simulink model "Mooventure2016_Rev5"  (Simulink 7.7)
settings: Solver=FixedStepDiscrete  StartTime=0.0  StopTime=10  RelTol=1e-3
PreLoadFcn:
  | try, eval([bdroot '_setup']); catch, eval('model_setup', ''); end
InitFcn:
  | try, eval([bdroot '_setup']); catch, eval('model_setup', ''); end
undefined symbols (not defined in the file): ECM, H1, motohawk_build_version, motohawk_trunc_name, motohawk_vardec_config_group, motohawk_vardec_path, xD
libraries: MotoHawk_lib x976, motohawk_control_primitives_lib x41, simulink x27, motohawk_annotations_lib x3
(part 13 of 16)

== system Mooventure2016_Rev5/Foreground/Control/Faults/Accesories/HV-Heater System ==
  In1 : Inport
  Abs : Abs
  Add : Sum
  Add1 : Sum  Inputs=+-
  Bus Selector : BusSelector  OutputSignals=Analog_Inputs.Coolant.temp_reading
  Bus Selector1 : BusSelector  OutputSignals=Analog_Inputs.Coolant.temp_reading
  Bus Selector2 : BusSelector  OutputSignals=Analog_Inputs.Coolant.Heater_Temp_Raw
  Bus Selector3 : BusSelector  OutputSignals=Analog_Inputs.Coolant.Heater_Temp_Raw
  Bus Selector4 : BusSelector  OutputSignals=Analog_Inputs.Coolant.Heater_Temp_Raw
  Logical Operator : Logic  Operator=OR  Inputs=4  AllPortsSameDT=off  OutDataTypeStr=boolean
  Logical Operator1 : Logic  Operator=NOT  AllPortsSameDT=off  OutDataTypeStr=boolean
  Logical Operator2 : Logic  AllPortsSameDT=off  OutDataTypeStr=boolean
  Relational Operator : RelationalOperator  OutDataTypeStr=boolean
  Relational Operator1 : RelationalOperator  Operator=>  OutDataTypeStr=boolean
  Relational Operator2 : RelationalOperator  OutDataTypeStr=boolean
  Relational Operator3 : RelationalOperator  Operator=<  OutDataTypeStr=boolean
  Relational Operator4 : RelationalOperator  Operator=>  OutDataTypeStr=boolean
  Triggered Subsystem : Subsystem  TreatAsAtomicUnit=on
  Unit Delay : UnitDelay  SampleTime=-1
  motohawk_calibration : MotoHawk_lib/Calibration & Probing Blocks/motohawk_calibration  nam='Temp_Fault_Hyst'  val=4  storage=Calibration  show_more=off  name_source=Use Parameter  data_type=Inherit from 'Default Value'  read_level=1  write_level=1  ovr_cals=on  view_as=Number  enum_struct={'Disabled', 'Enabled'}  vector_style=Wide Row  use_help_units=off  help=''  units=''  use_header_enum=off  row_header_enum={}  col_header_enum={}  use_min_max=off  min_val=-inf  max_val=inf  use_precision=off  precision=''  gain=1  offset=0  exp=1  use_mototune_group=off  mototune_group=motohawk_vardec_path(gcb)
  motohawk_calibration1 : MotoHawk_lib/Calibration & Probing Blocks/motohawk_calibration  nam='HV_Heater_Over_Temperature_Fault'  val=93  storage=Calibration  show_more=off  name_source=Use Parameter  data_type=Inherit from 'Default Value'  read_level=1  write_level=1  ovr_cals=on  view_as=Number  enum_struct={'Disabled', 'Enabled'}  vector_style=Wide Row  use_help_units=off  help=''  units=''  use_header_enum=off  row_header_enum={}  col_header_enum={}  use_min_max=off  min_val=-inf  max_val=inf  use_precision=off  precision=''  gain=1  offset=0  exp=1  use_mototune_group=off  mototune_group=motohawk_vardec_path(gcb)
  motohawk_calibration2 : MotoHawk_lib/Calibration & Probing Blocks/motohawk_calibration  nam='HV_Heater_Temperature_Sensor_A_Intermittent_Fault'  val=4  storage=Calibration  show_more=off  name_source=Use Parameter  data_type=Inherit from 'Default Value'  read_level=1  write_level=1  ovr_cals=on  view_as=Number  enum_struct={'Disabled', 'Enabled'}  vector_style=Wide Row  use_help_units=off  help=''  units=''  use_header_enum=off  row_header_enum={}  col_header_enum={}  use_min_max=off  min_val=-inf  max_val=inf  use_precision=off  precision=''  gain=1  offset=0  exp=1  use_mototune_group=off  mototune_group=motohawk_vardec_path(gcb)
  motohawk_calibration3 : MotoHawk_lib/Calibration & Probing Blocks/motohawk_calibration  nam='HV_Heater_Temperature_Sensor_A_Low_Voltage_Fault'  val=20  storage=Calibration  show_more=off  name_source=Use Parameter  data_type=Inherit from 'Default Value'  read_level=1  write_level=1  ovr_cals=on  view_as=Number  enum_struct={'Disabled', 'Enabled'}  vector_style=Wide Row  use_help_units=off  help=''  units=''  use_header_enum=off  row_header_enum={}  col_header_enum={}  use_min_max=off  min_val=-inf  max_val=inf  use_precision=off  precision=''  gain=1  offset=0  exp=1  use_mototune_group=off  mototune_group=motohawk_vardec_path(gcb)
  motohawk_calibration4 : MotoHawk_lib/Calibration & Probing Blocks/motohawk_calibration  nam='HV_Heater_Temperature_Sensor_A_High_Voltage_Fault'  val=250  storage=Calibration  show_more=off  name_source=Use Parameter  data_type=Inherit from 'Default Value'  read_level=1  write_level=1  ovr_cals=on  view_as=Number  enum_struct={'Disabled', 'Enabled'}  vector_style=Wide Row  use_help_units=off  help=''  units=''  use_header_enum=off  row_header_enum={}  col_header_enum={}  use_min_max=off  min_val=-inf  max_val=inf  use_precision=off  precision=''  gain=1  offset=0  exp=1  use_mototune_group=off  mototune_group=motohawk_vardec_path(gcb)
  motohawk_data_def : MotoHawk_lib/Data Storage Blocks/motohawk_data_def  nam='TempReading'  container_nam=''  data=23  typ=double  struct_nam='MyStruct'  storage=Volatile  outputRef=off  use_vardec=off  window=Display  read_level=1  write_level=1  ovr_cals=on  view_as=Number  enum_struct={'Disabled', 'Enabled'}  vector_style=Wide Row  use_help_units=off  help=''  units=''  use_header_enum=off  row_header_enum=''  col_header_enum=''  use_min_max=off  min_val=-inf  max_val=inf  use_precision=off  precision=''  gain=1  offset=0  exp=1  use_mototune_group=off  mototune_group=motohawk_vardec_path(gcb)  eval_name=MyData  data_stores=motohawk_sfun_data_def_data_stores  struct_instances=motohawk_sfun_data_def_struct_instances  vardecs=motohawk_sfun_data_def_vardecs
  motohawk_data_read : MotoHawk_lib/Data Storage Blocks/motohawk_data_read  source=Lookup By Name  structure=Scalar  operation=Read scalar from location by index  sz_vec=4  sz_row=2  sz_col=3  typ=double  nam='TempReading'  checkNull=on  struct_inst_name='MyData'  struct_nam='MyStruct'
  motohawk_fault_def1 : MotoHawk_lib/Fault Management Blocks/motohawk_fault_def  nam='HV_Heater_Poor_Performance'  mode=Enabled  id=['B1B30']  x=1500  y=2000  input_suspected=on  indeterminate=off  increment_xy=on  downsample_count=1  ovr_cals=on  ovr_actions=on  show_actions=on  action1_name=''  action1_cond=(None)  action2_name=''  action2_cond=(None)  action3_name=''  action3_cond=(None)  action4_name=''  action4_cond=(None)
  motohawk_fault_def2 : MotoHawk_lib/Fault Management Blocks/motohawk_fault_def  nam='HV_Heater_Over_Temperature'  mode=Enabled  id=['B1B31']  x=9  y=10  input_suspected=on  indeterminate=off  increment_xy=on  downsample_count=1  ovr_cals=on  ovr_actions=on  show_actions=on  action1_name=''  action1_cond=(None)  action2_name=''  action2_cond=(None)  action3_name=''  action3_cond=(None)  action4_name=''  action4_cond=(None)
  motohawk_fault_def3 : MotoHawk_lib/Fault Management Blocks/motohawk_fault_def  nam='HV_Heater_Temperature_Sensor_A_Intermittent'  mode=Enabled  id=['B1B32']  x=9  y=10  input_suspected=on  indeterminate=off  increment_xy=on  downsample_count=1  ovr_cals=on  ovr_actions=on  show_actions=on  action1_name=''  action1_cond=(None)  action2_name=''  action2_cond=(None)  action3_name=''  action3_cond=(None)  action4_name=''  action4_cond=(None)
  motohawk_fault_def4 : MotoHawk_lib/Fault Management Blocks/motohawk_fault_def  nam='HV_Heater_Temperature_Sensor_A_Low_Voltage'  mode=Enabled  id=['B1B33']  x=9  y=10  input_suspected=on  indeterminate=off  increment_xy=on  downsample_count=1  ovr_cals=on  ovr_actions=on  show_actions=on  action1_name=''  action1_cond=(None)  action2_name=''  action2_cond=(None)  action3_name=''  action3_cond=(None)  action4_name=''  action4_cond=(None)
  motohawk_fault_def5 : MotoHawk_lib/Fault Management Blocks/motohawk_fault_def  nam='HV_Heater_Temperature_Sensor_A_High_Voltage'  mode=Enabled  id=['B1B34']  x=9  y=10  input_suspected=on  indeterminate=off  increment_xy=on  downsample_count=1  ovr_cals=on  ovr_actions=on  show_actions=on  action1_name=''  action1_cond=(None)  action2_name=''  action2_cond=(None)  action3_name=''  action3_cond=(None)  action4_name=''  action4_cond=(None)
  wires:
  In1/1 -> Bus Selector/1, Bus Selector1/1, Bus Selector2/1, Bus Selector3/1, Bus Selector4/1
  [Heat1] -> Logical Operator/1
  [Heat2] -> Logical Operator/2
  [Heat3] -> Logical Operator/3
  [Heat4] -> Logical Operator/4
  Bus Selector/1 -> Triggered Subsystem/1(In1), Add/2  "<temp_reading>"
  Logical Operator/1 -> Triggered Subsystem/Trigger, Logical Operator2/2
  motohawk_calibration/1 -> Add/1
  Add/1 -> Relational Operator/1
  motohawk_data_read/1 -> Relational Operator/2
  Relational Operator/1 -> Logical Operator1/1
  Logical Operator1/1 -> Logical Operator2/1
  Logical Operator2/1 -> motohawk_fault_def1/1
  motohawk_calibration1/1 -> Relational Operator1/2
  Relational Operator1/1 -> motohawk_fault_def2/1
  Bus Selector1/1 -> Relational Operator1/1  "<temp_reading>"
  Bus Selector2/1 -> Add1/1, Unit Delay/1  "<Heater_Temp_Raw>"
  Unit Delay/1 -> Add1/2
  Add1/1 -> Abs/1
  Abs/1 -> Relational Operator2/1
  Relational Operator2/1 -> motohawk_fault_def3/1
  motohawk_calibration2/1 -> Relational Operator2/2
  motohawk_calibration3/1 -> Relational Operator3/2
  Relational Operator3/1 -> motohawk_fault_def4/1
  Bus Selector3/1 -> Relational Operator3/1  "<Heater_Temp_Raw>"
  motohawk_calibration4/1 -> Relational Operator4/2
  Relational Operator4/1 -> motohawk_fault_def5/1
  Bus Selector4/1 -> Relational Operator4/1  "<Heater_Temp_Raw>"

== system Mooventure2016_Rev5/Foreground/Control/Faults/Battery/2G BMS & Comms ==
  In1 : Inport
  Add : Sum  Inputs=+-
  Bus Selector1 : BusSelector  OutputSignals=Battery_Inputs.CellBalanceingActive
  Bus Selector2 : BusSelector  OutputSignals=Battery_Inputs.ActiveDTC
  Bus Selector3 : BusSelector  OutputSignals=Battery_Inputs.BatteryCurrent
  Bus Selector4 : BusSelector  OutputSignals=Battery_Inputs.AgeCount
  Bus Selector5 : BusSelector  OutputSignals=Battery_Inputs.MaxCellVoltage,Battery_Inputs.MinCellVoltage
  Bus Selector6 : BusSelector  OutputSignals=Battery_Inputs.StateOfCharge
  Bus Selector7 : BusSelector  OutputSignals=Battery_Inputs.BatteryVoltage
  Logical Operator : Logic  AllPortsSameDT=off  OutDataTypeStr=boolean
  Relational Operator{1..3,6} (4 alike) : RelationalOperator  Operator=>  OutDataTypeStr=boolean
  Relational Operator4 : RelationalOperator  OutDataTypeStr=boolean
  Relational Operator5 : RelationalOperator  Operator===  OutDataTypeStr=boolean
  motohawk_calibration1 : MotoHawk_lib/Calibration & Probing Blocks/motohawk_calibration  nam='HV_Battery_2G_BMS_Fault'  val=0  storage=Calibration  show_more=off  name_source=Use Parameter  data_type=Inherit from 'Default Value'  read_level=1  write_level=1  ovr_cals=on  view_as=Number  enum_struct={'Disabled', 'Enabled'}  vector_style=Wide Row  use_help_units=off  help=''  units=''  use_header_enum=off  row_header_enum={}  col_header_enum={}  use_min_max=off  min_val=-inf  max_val=inf  use_precision=off  precision=''  gain=1  offset=0  exp=1  use_mototune_group=off  mototune_group=motohawk_vardec_path(gcb)
  motohawk_calibration2 : MotoHawk_lib/Calibration & Probing Blocks/motohawk_calibration  nam='HV_Battery_Cell_Balancing_Required_Fault'  val=0.3  storage=Calibration  show_more=off  name_source=Use Parameter  data_type=Inherit from 'Default Value'  read_level=1  write_level=1  ovr_cals=on  view_as=Number  enum_struct={'Disabled', 'Enabled'}  vector_style=Wide Row  use_help_units=off  help=''  units=''  use_header_enum=off  row_header_enum={}  col_header_enum={}  use_min_max=off  min_val=-inf  max_val=inf  use_precision=off  precision=''  gain=1  offset=0  exp=1  use_mototune_group=off  mototune_group=motohawk_vardec_path(gcb)
  motohawk_calibration3 : MotoHawk_lib/Calibration & Probing Blocks/motohawk_calibration  nam='HV_Battery_Try_To_Balance_Under_Load_Fault'  val=1  storage=Calibration  show_more=off  name_source=Use Parameter  data_type=Inherit from 'Default Value'  read_level=1  write_level=1  ovr_cals=on  view_as=Number  enum_struct={'Disabled', 'Enabled'}  vector_style=Wide Row  use_help_units=off  help=''  units=''  use_header_enum=off  row_header_enum={}  col_header_enum={}  use_min_max=off  min_val=-inf  max_val=inf  use_precision=off  precision=''  gain=1  offset=0  exp=1  use_mototune_group=off  mototune_group=motohawk_vardec_path(gcb)
  motohawk_calibration4 : MotoHawk_lib/Calibration & Probing Blocks/motohawk_calibration  nam='HV_Battery_48_Controller_Communication_Fault'  val=1000  storage=Calibration  show_more=off  name_source=Use Parameter  data_type=Inherit from 'Default Value'  read_level=1  write_level=1  ovr_cals=on  view_as=Number  enum_struct={'Disabled', 'Enabled'}  vector_style=Wide Row  use_help_units=off  help=''  units=''  use_header_enum=off  row_header_enum={}  col_header_enum={}  use_min_max=off  min_val=-inf  max_val=inf  use_precision=off  precision=''  gain=1  offset=0  exp=1  use_mototune_group=off  mototune_group=motohawk_vardec_path(gcb)
  motohawk_calibration5 : MotoHawk_lib/Calibration & Probing Blocks/motohawk_calibration  nam='HV_Battery_Too_Low_For_Load_Fault'  val=0  storage=Calibration  show_more=off  name_source=Use Parameter  data_type=Inherit from 'Default Value'  read_level=1  write_level=1  ovr_cals=on  view_as=Number  enum_struct={'Disabled', 'Enabled'}  vector_style=Wide Row  use_help_units=off  help=''  units=''  use_header_enum=off  row_header_enum={}  col_header_enum={}  use_min_max=off  min_val=-inf  max_val=inf  use_precision=off  precision=''  gain=1  offset=0  exp=1  use_mototune_group=off  mototune_group=motohawk_vardec_path(gcb)
  motohawk_calibration6 : MotoHawk_lib/Calibration & Probing Blocks/motohawk_calibration  nam='HV_Battery_Above_Safe_Charge_Point'  val=395  storage=Calibration  show_more=off  name_source=Use Parameter  data_type=Inherit from 'Default Value'  read_level=1  write_level=1  ovr_cals=on  view_as=Number  enum_struct={'Disabled', 'Enabled'}  vector_style=Wide Row  use_help_units=off  help=''  units=''  use_header_enum=off  row_header_enum={}  col_header_enum={}  use_min_max=off  min_val=-inf  max_val=inf  use_precision=off  precision=''  gain=1  offset=0  exp=1  use_mototune_group=off  mototune_group=motohawk_vardec_path(gcb)
  motohawk_fault_def1 : MotoHawk_lib/Fault Management Blocks/motohawk_fault_def  nam='HV_Battery_2G_BMS_Fault'  mode=Enabled  id=['B1C47']  x=9  y=10  input_suspected=on  indeterminate=off  increment_xy=on  downsample_count=1  ovr_cals=on  ovr_actions=on  show_actions=on  action1_name='HV_Light'  action1_cond=Active  action2_name=''  action2_cond=(None)  action3_name=''  action3_cond=(None)  action4_name=''  action4_cond=(None)
  motohawk_fault_def2 : MotoHawk_lib/Fault Management Blocks/motohawk_fault_def  nam='HV_Battery_Too_Low_For_Load'  mode=Enabled  id=['B1C4A']  x=1500  y=2000  input_suspected=on  indeterminate=off  increment_xy=on  downsample_count=1  ovr_cals=on  ovr_actions=on  show_actions=on  action1_name='HV_Light'  action1_cond=Active  action2_name=''  action2_cond=(None)  action3_name=''  action3_cond=(None)  action4_name=''  action4_cond=(None)
  motohawk_fault_def3 : MotoHawk_lib/Fault Management Blocks/motohawk_fault_def  nam='HV_Battery_Try_To_Balance_Under_Load'  mode=Enabled  id=['B1C48']  x=9  y=10  input_suspected=on  indeterminate=off  increment_xy=on  downsample_count=1  ovr_cals=on  ovr_actions=on  show_actions=on  action1_name=''  action1_cond=(None)  action2_name=''  action2_cond=(None)  action3_name=''  action3_cond=(None)  action4_name=''  action4_cond=(None)
  motohawk_fault_def4 : MotoHawk_lib/Fault Management Blocks/motohawk_fault_def  nam='HV_Battery_Cell_Balancing_Required_Fault'  mode=Disabled  id=['B1C49']  x=9  y=10  input_suspected=on  indeterminate=off  increment_xy=on  downsample_count=1  ovr_cals=on  ovr_actions=on  show_actions=on  action1_name='HV_Light'  action1_cond=Active  action2_name=''  action2_cond=(None)  action3_name=''  action3_cond=(None)  action4_name=''  action4_cond=(None)
  motohawk_fault_def5 : MotoHawk_lib/Fault Management Blocks/motohawk_fault_def  nam='HV_Battery_48_Controller_Communication_Fault'  mode=Enabled  id=['B1C50']  x=5  y=10  input_suspected=on  indeterminate=off  increment_xy=on  downsample_count=1  ovr_cals=on  ovr_actions=on  show_actions=on  action1_name='HV_Light'  action1_cond=Active  action2_name='Dyno_Shutdown'  action2_cond=Active  action3_name=''  action3_cond=(None)  action4_name=''  action4_cond=(None)
  motohawk_fault_def6 : MotoHawk_lib/Fault Management Blocks/motohawk_fault_def  nam='HV_Battery_Above_Safe_Charge_Point'  mode=Enabled  id=['B1C4B']  x=1500  y=2000  input_suspected=on  indeterminate=off  increment_xy=on  downsample_count=1  ovr_cals=on  ovr_actions=on  show_actions=on  action1_name='HV_Light'  action1_cond=Active  action2_name='Dyno_Shutdown'  action2_cond=Active  action3_name=''  action3_cond=(None)  action4_name=''  action4_cond=(None)
  wires:
  Bus Selector4/1 -> Relational Operator4/1  "<AgeCount>"
  motohawk_calibration4/1 -> Relational Operator4/2
  Relational Operator4/1 -> motohawk_fault_def5/1
  In1/1 -> Bus Selector4/1, Bus Selector2/1, Bus Selector3/1, Bus Selector1/1, Bus Selector5/1, Bus Selector6/1, Bus Selector7/1
  motohawk_calibration1/1 -> Relational Operator1/2
  Relational Operator1/1 -> motohawk_fault_def1/1
  Bus Selector2/1 -> Relational Operator1/1  "<ActiveDTC>"
  motohawk_calibration3/1 -> Relational Operator3/2
  Bus Selector3/1 -> Relational Operator3/1  "<BatteryCurrent>"
  Relational Operator3/1 -> Logical Operator/1
  Logical Operator/1 -> motohawk_fault_def3/1
  Bus Selector1/1 -> Logical Operator/2  "<CellBalanceingActive>"
  Bus Selector5/1 -> Add/1  "<MaxCellVoltage>"
  Bus Selector5/2 -> Add/2  "<MinCellVoltage>"
  motohawk_calibration2/1 -> Relational Operator2/2
  Add/1 -> Relational Operator2/1  "<BatteryCurrent>"
  Relational Operator2/1 -> motohawk_fault_def4/1
  motohawk_calibration5/1 -> Relational Operator5/2
  Relational Operator5/1 -> motohawk_fault_def2/1
  Bus Selector6/1 -> Relational Operator5/1  "<StateOfCharge>"
  motohawk_calibration6/1 -> Relational Operator6/2
  Relational Operator6/1 -> motohawk_fault_def6/1
  Bus Selector7/1 -> Relational Operator6/1  "<BatteryVoltage>"

== system Mooventure2016_Rev5/Foreground/Control/Faults/Battery/Precharge ==
  In1 : Inport
  Bus Selector1 : BusSelector  OutputSignals=Battery_Inputs.PrechargeState
  Relational Operator2 : RelationalOperator  Operator===  OutDataTypeStr=boolean
  motohawk_calibration2 : MotoHawk_lib/Calibration & Probing Blocks/motohawk_calibration  nam='HV_Battery_Precharge_Failure_Fault'  val=4  storage=Calibration  show_more=off  name_source=Use Parameter  data_type=Inherit from 'Default Value'  read_level=1  write_level=1  ovr_cals=on  view_as=Number  enum_struct={'Disabled', 'Enabled'}  vector_style=Wide Row  use_help_units=off  help=''  units=''  use_header_enum=off  row_header_enum={}  col_header_enum={}  use_min_max=off  min_val=-inf  max_val=inf  use_precision=off  precision=''  gain=1  offset=0  exp=1  use_mototune_group=off  mototune_group=motohawk_vardec_path(gcb)
  motohawk_fault_def2 : MotoHawk_lib/Fault Management Blocks/motohawk_fault_def  nam='HV_Battery_Precharge_Failure'  mode=Enabled  id=['B1C42']  x=9  y=10  input_suspected=on  indeterminate=off  increment_xy=on  downsample_count=1  ovr_cals=on  ovr_actions=on  show_actions=on  action1_name='HV_Light'  action1_cond=Active  action2_name=''  action2_cond=(None)  action3_name=''  action3_cond=(None)  action4_name=''  action4_cond=(None)
  wires:
  motohawk_calibration2/1 -> Relational Operator2/2
  Relational Operator2/1 -> motohawk_fault_def2/1
  Bus Selector1/1 -> Relational Operator2/1  "<PrechargeState>"
  In1/1 -> Bus Selector1/1

== system Mooventure2016_Rev5/Foreground/Control/Faults/Battery/Temperature ==
  In1 : Inport
  Bus Selector : BusSelector  OutputSignals=Battery_Inputs.MinCellTemperature
  Bus Selector1 : BusSelector  OutputSignals=Battery_Inputs.MinCellTemperature
  Bus Selector2 : BusSelector  OutputSignals=Battery_Inputs.MaxCellTemperature
  Bus Selector3 : BusSelector  OutputSignals=Battery_Inputs.MaxCellTemperature
  Logical Operator : Logic  AllPortsSameDT=off  OutDataTypeStr=boolean
  Logical Operator1 : Logic  AllPortsSameDT=off  OutDataTypeStr=boolean
  Relational Operator1 : RelationalOperator  Operator=>  OutDataTypeStr=boolean
  Relational Operator2 : RelationalOperator  Operator=<=  OutDataTypeStr=boolean
  Relational Operator3 : RelationalOperator  Operator=>  OutDataTypeStr=boolean
  Relational Operator4 : RelationalOperator  Operator=<=  OutDataTypeStr=boolean
  Relational Operator6 : RelationalOperator  Operator=>  OutDataTypeStr=boolean
  Relational Operator7 : RelationalOperator  Operator=<=  OutDataTypeStr=boolean
  motohawk_calibration1 : MotoHawk_lib/Calibration & Probing Blocks/motohawk_calibration  nam='HV_Battery_Pack_Above_Operating_Temperature_Fault'  val=50  storage=Calibration  show_more=off  name_source=Use Parameter  data_type=Inherit from 'Default Value'  read_level=1  write_level=1  ovr_cals=on  view_as=Number  enum_struct={'Disabled', 'Enabled'}  vector_style=Wide Row  use_help_units=off  help=''  units=''  use_header_enum=off  row_header_enum={}  col_header_enum={}  use_min_max=off  min_val=-inf  max_val=inf  use_precision=off  precision=''  gain=1  offset=0  exp=1  use_mototune_group=off  mototune_group=motohawk_vardec_path(gcb)
  motohawk_calibration2 : MotoHawk_lib/Calibration & Probing Blocks/motohawk_calibration  nam='HV_Battery_Pack_Below_Operating_Temperature_Fault'  val=-20  storage=Calibration  show_more=off  name_source=Use Parameter  data_type=Inherit from 'Default Value'  read_level=1  write_level=1  ovr_cals=on  view_as=Number  enum_struct={'Disabled', 'Enabled'}  vector_style=Wide Row  use_help_units=off  help=''  units=''  use_header_enum=off  row_header_enum={}  col_header_enum={}  use_min_max=off  min_val=-inf  max_val=inf  use_precision=off  precision=''  gain=1  offset=0  exp=1  use_mototune_group=off  mototune_group=motohawk_vardec_path(gcb)
  motohawk_calibration3 : MotoHawk_lib/Calibration & Probing Blocks/motohawk_calibration  nam='HV_Battery_Pack_Low_Temperature_Fault_Low'  val=-20  storage=Calibration  show_more=off  name_source=Use Parameter  data_type=Inherit from 'Default Value'  read_level=1  write_level=1  ovr_cals=on  view_as=Number  enum_struct={'Disabled', 'Enabled'}  vector_style=Wide Row  use_help_units=off  help=''  units=''  use_header_enum=off  row_header_enum={}  col_header_enum={}  use_min_max=off  min_val=-inf  max_val=inf  use_precision=off  precision=''  gain=1  offset=0  exp=1  use_mototune_group=off  mototune_group=motohawk_vardec_path(gcb)
  motohawk_calibration4 : MotoHawk_lib/Calibration & Probing Blocks/motohawk_calibration  nam='HV_Battery_Pack_Low_Temperature_Fault_High'  val=-10  storage=Calibration  show_more=off  name_source=Use Parameter  data_type=Inherit from 'Default Value'  read_level=1  write_level=1  ovr_cals=on  view_as=Number  enum_struct={'Disabled', 'Enabled'}  vector_style=Wide Row  use_help_units=off  help=''  units=''  use_header_enum=off  row_header_enum={}  col_header_enum={}  use_min_max=off  min_val=-inf  max_val=inf  use_precision=off  precision=''  gain=1  offset=0  exp=1  use_mototune_group=off  mototune_group=motohawk_vardec_path(gcb)
  motohawk_calibration5 : MotoHawk_lib/Calibration & Probing Blocks/motohawk_calibration  nam='HV_Battery_Pack_High_Temperature_Fault_Low'  val=40  storage=Calibration  show_more=off  name_source=Use Parameter  data_type=Inherit from 'Default Value'  read_level=1  write_level=1  ovr_cals=on  view_as=Number  enum_struct={'Disabled', 'Enabled'}  vector_style=Wide Row  use_help_units=off  help=''  units=''  use_header_enum=off  row_header_enum={}  col_header_enum={}  use_min_max=off  min_val=-inf  max_val=inf  use_precision=off  precision=''  gain=1  offset=0  exp=1  use_mototune_group=off  mototune_group=motohawk_vardec_path(gcb)
  motohawk_calibration6 : MotoHawk_lib/Calibration & Probing Blocks/motohawk_calibration  nam='HV_Battery_Pack_High_Temperature_Fault_High'  val=50  storage=Calibration  show_more=off  name_source=Use Parameter  data_type=Inherit from 'Default Value'  read_level=1  write_level=1  ovr_cals=on  view_as=Number  enum_struct={'Disabled', 'Enabled'}  vector_style=Wide Row  use_help_units=off  help=''  units=''  use_header_enum=off  row_header_enum={}  col_header_enum={}  use_min_max=off  min_val=-inf  max_val=inf  use_precision=off  precision=''  gain=1  offset=0  exp=1  use_mototune_group=off  mototune_group=motohawk_vardec_path(gcb)
  motohawk_fault_def1 : MotoHawk_lib/Fault Management Blocks/motohawk_fault_def  nam='HV_Battery_Pack_Low_Temperature'  mode=Enabled  id=['B1C10']  x=9  y=10  input_suspected=on  indeterminate=off  increment_xy=on  downsample_count=1  ovr_cals=on  ovr_actions=on  show_actions=on  action1_name='Temperature_Flash'  action1_cond=Active  action2_name=''  action2_cond=(None)  action3_name=''  action3_cond=(None)  action4_name=''  action4_cond=(None)
  motohawk_fault_def2 : MotoHawk_lib/Fault Management Blocks/motohawk_fault_def  nam='HV_Battery_Pack_Below_Operating_Temperature'  mode=Enabled  id=['B1C11']  x=9  y=10  input_suspected=on  indeterminate=off  increment_xy=on  downsample_count=1  ovr_cals=on  ovr_actions=on  show_actions=on  action1_name='Temperature_Flash'  action1_cond=Active  action2_name='HV_Light'  action2_cond=Active  action3_name=''  action3_cond=(None)  action4_name=''  action4_cond=(None)
  motohawk_fault_def3 : MotoHawk_lib/Fault Management Blocks/motohawk_fault_def  nam='HV_Battery_Pack_High_Temperature'  mode=Enabled  id=['B1C12']  x=9  y=10  input_suspected=on  indeterminate=off  increment_xy=on  downsample_count=1  ovr_cals=on  ovr_actions=on  show_actions=on  action1_name='Temperature_Flash'  action1_cond=Active  action2_name='Cooling_Max'  action2_cond=Active  action3_name=''  action3_cond=(None)  action4_name=''  action4_cond=(None)
  motohawk_fault_def4 : MotoHawk_lib/Fault Management Blocks/motohawk_fault_def  nam='HV_Battery_Pack_Above_Operating_Temperature'  mode=Enabled  id=['B1C13']  x=9  y=10  input_suspected=on  indeterminate=off  increment_xy=on  downsample_count=1  ovr_cals=on  ovr_actions=on  show_actions=on  action1_name='Temperature_Flash'  action1_cond=Active  action2_name='HV_Light'  action2_cond=Active  action3_name='Cooling_Max'  action3_cond=Active  action4_name=''  action4_cond=(None)
  wires:
  In1/1 -> Bus Selector/1, Bus Selector1/1, Bus Selector2/1, Bus Selector3/1
  motohawk_calibration2/1 -> Relational Operator2/2
  Relational Operator2/1 -> motohawk_fault_def2/1
  Bus Selector1/1 -> Relational Operator2/1  "<MinCellTemperature>"
  motohawk_calibration3/1 -> Relational Operator6/2
  Relational Operator7/1 -> Logical Operator/2
  Relational Operator6/1 -> Logical Operator/1
  Logical Operator/1 -> motohawk_fault_def1/1
  motohawk_calibration4/1 -> Relational Operator7/2
  Bus Selector/1 -> Relational Operator6/1, Relational Operator7/1  "<MinCellTemperature>"
  motohawk_calibration1/1 -> Relational Operator1/2
  Relational Operator1/1 -> motohawk_fault_def4/1
  Bus Selector3/1 -> Relational Operator1/1  "<MaxCellTemperature>"
  motohawk_calibration5/1 -> Relational Operator3/2
  Relational Operator4/1 -> Logical Operator1/2
  Relational Operator3/1 -> Logical Operator1/1
  Logical Operator1/1 -> motohawk_fault_def3/1
  motohawk_calibration6/1 -> Relational Operator4/2
  Bus Selector2/1 -> Relational Operator3/1, Relational Operator4/1  "<MaxCellTemperature>"

== system Mooventure2016_Rev5/Foreground/Control/Faults/Freeze Frame/Data Write ==
  In1 : Inport
  Trigger : TriggerPort  TriggerType=function-call
  Bus Creator : BusCreator  Inputs=6
  Bus Selector : BusSelector  OutputSignals=IPT.ID 278 IPT Status 1.IPT_HVDCVoltage,IPT.ID 260 IPT Status 2.IPT_MotorSpeed
  Bus Selector1 : BusSelector  OutputSignals=IPT.ID 260 IPT Status 2.IPT_WheelTorqueDelivered,IPT.ID 278 IPT Status 1.IPT_InverterTemperature
  Data Iterator : Stateflow chart  TreatAsAtomicUnit=on
  motohawk_abs_time : MotoHawk_lib/Extra Development Blocks/motohawk_abs_time  mode=Seconds (double)
  motohawk_data_read : MotoHawk_lib/Data Storage Blocks/motohawk_data_read  source=Lookup By Name  structure=Scalar  operation=Read scalar from location by index  sz_vec=4  sz_row=2  sz_col=3  typ=double  nam='TorqueRequest'  checkNull=on  struct_inst_name='MyData'  struct_nam='MyStruct'
  motohawk_data_sizeof : MotoHawk_lib/Data Storage Blocks/motohawk_data_sizeof  source=Lookup By Name  out_format=Rows  dt=uint32  nam='Freeze_Frame'  struct_inst_name='Fault1_'
  motohawk_data_write : MotoHawk_lib/Data Storage Blocks/motohawk_data_write  source=Lookup By Name  structure=Matrix  operation=Write scalar into location by index  sz_vec=9  sz_row=2  sz_col=9  typ=double  nam='Freeze_Frame'  checkNull=on  write_read_only=off  struct_inst_name=''  struct_name='MyStruct'
  wires:
  Data Iterator/2(row) -> motohawk_data_write/2
  Data Iterator/3(col) -> motohawk_data_write/3
  motohawk_data_sizeof/1 -> Data Iterator/2(currentRow)
  In1/1 -> Bus Selector/1, Bus Selector1/1
  motohawk_abs_time/1 -> Bus Creator/1
  Bus Selector/1 -> Bus Creator/2  "<IPT_HVDCVoltage>"
  Bus Selector/2 -> Bus Creator/3  "<IPT_MotorSpeed>"
  Bus Selector1/1 -> Bus Creator/5  "<IPT_WheelTorqueDelivered>"
  Bus Selector1/2 -> Bus Creator/6  "<IPT_InverterTemperature>"
  Bus Creator/1 -> Data Iterator/1(dataIn)  "dataIn"
  Data Iterator/1(data) -> motohawk_data_write/1
  motohawk_data_read/1 -> Bus Creator/4  "Torque_Request"

== system Mooventure2016_Rev5/Foreground/Control/Faults/Power Train/12V Battery ==
  Abs : Abs
  Add : Sum  Inputs=+-
  Constant : Constant  Value=.02697
  Logical Operator2 : Logic  Operator=OR  Inputs=3  AllPortsSameDT=off  OutDataTypeStr=boolean
  Product : Product  RndMeth=Zero
  Relational Operator : RelationalOperator  OutDataTypeStr=boolean
  Relational Operator1 : RelationalOperator  Operator=<=  OutDataTypeStr=boolean
  Relational Operator2 : RelationalOperator  OutDataTypeStr=boolean
  Unit Delay : UnitDelay  SampleTime=-1
  motohawk_ain : MotoHawk_lib/Analog I//O Blocks/motohawk_ain  res_name=[]  text_resource=DRVP  code_resource=NONE  val_resource=-1  target=ECM-5554-112-0904-xD  resource_enum_str=(None)=-1,AN24=1,AN25=2,AN26=3,AN27=4,AN28=5,AN29=6,AN30=7,AN31=8,AN32=9,AN33=10,ECUP=11,ESTOP=12,DRVP=13,XDRP=14,XDRP_B=15,AN1=16,AN2=17,AN3=18,AN4=19,AN5=20,AN6=21,AN7=22,AN8=23,AN9=24,AN10=25,AN11=26,AN12=27,AN13=28,AN14=29,AN15=30,AN16=31,AN17=32,AN18=33,AN19=34,AN20=35,AN21=36,AN22=37,AN23=38,O2A=39,O2B=40,O2C=41,O2D=42  altref=5V Reference  typ=uint16  num_adc_bits=10  use_stat=off  use_vardec=off  nam='RTD1_MW'  read_level=1  write_level=1  group='System | I/O Pins | Inputs Config'
  motohawk_calibration1 : MotoHawk_lib/Calibration & Probing Blocks/motohawk_calibration  nam='V12_Low'  val=12  storage=Calibration  show_more=off  name_source=Use Parameter  data_type=Inherit from 'Default Value'  read_level=1  write_level=1  ovr_cals=on  view_as=Number  enum_struct={'Disabled', 'Enabled'}  vector_style=Wide Row  use_help_units=off  help=''  units=''  use_header_enum=off  row_header_enum={}  col_header_enum={}  use_min_max=off  min_val=-inf  max_val=inf  use_precision=off  precision=''  gain=1  offset=0  exp=1  use_mototune_group=off  mototune_group=motohawk_vardec_path(gcb)
  motohawk_calibration2 : MotoHawk_lib/Calibration & Probing Blocks/motohawk_calibration  nam='V12_High'  val=14.2  storage=Calibration  show_more=off  name_source=Use Parameter  data_type=Inherit from 'Default Value'  read_level=1  write_level=1  ovr_cals=on  view_as=Number  enum_struct={'Disabled', 'Enabled'}  vector_style=Wide Row  use_help_units=off  help=''  units=''  use_header_enum=off  row_header_enum={}  col_header_enum={}  use_min_max=off  min_val=-inf  max_val=inf  use_precision=off  precision=''  gain=1  offset=0  exp=1  use_mototune_group=off  mototune_group=motohawk_vardec_path(gcb)
  motohawk_calibration4 : MotoHawk_lib/Calibration & Probing Blocks/motohawk_calibration  nam='V12_Battery_Erratic_Fault'  val=2  storage=Calibration  show_more=off  name_source=Use Parameter  data_type=Inherit from 'Default Value'  read_level=1  write_level=1  ovr_cals=on  view_as=Number  enum_struct={'Disabled', 'Enabled'}  vector_style=Wide Row  use_help_units=off  help=''  units=''  use_header_enum=off  row_header_enum={}  col_header_enum={}  use_min_max=off  min_val=-inf  max_val=inf  use_precision=off  precision=''  gain=1  offset=0  exp=1  use_mototune_group=off  mototune_group=motohawk_vardec_path(gcb)
  motohawk_fault_def1 : MotoHawk_lib/Fault Management Blocks/motohawk_fault_def  nam='System_Voltage_Low'  mode=Enabled  id=['P0562']  x=150  y=200  input_suspected=on  indeterminate=off  increment_xy=on  downsample_count=1  ovr_cals=on  ovr_actions=on  show_actions=on  action1_name='Batt_Light'  action1_cond=Active  action2_name=''  action2_cond=(None)  action3_name=''  action3_cond=(None)  action4_name=''  action4_cond=(None)
  motohawk_fault_def2 : MotoHawk_lib/Fault Management Blocks/motohawk_fault_def  nam='System_Voltage_Unstable'  mode=Enabled  id=['P0561']  x=9  y=10  input_suspected=on  indeterminate=off  increment_xy=on  downsample_count=1  ovr_cals=on  ovr_actions=on  show_actions=on  action1_name='Batt_Light'  action1_cond=Active  action2_name=''  action2_cond=(None)  action3_name=''  action3_cond=(None)  action4_name=''  action4_cond=(None)
  motohawk_fault_def3 : MotoHawk_lib/Fault Management Blocks/motohawk_fault_def  nam='System_Voltage_High'  mode=Enabled  id=['P0563']  x=150  y=200  input_suspected=on  indeterminate=off  increment_xy=on  downsample_count=1  ovr_cals=on  ovr_actions=on  show_actions=on  action1_name='Batt_Light'  action1_cond=Active  action2_name=''  action2_cond=(None)  action3_name=''  action3_cond=(None)  action4_name=''  action4_cond=(None)
  motohawk_fault_def4 : MotoHawk_lib/Fault Management Blocks/motohawk_fault_def  nam='System_Voltage_Malfunction'  mode=Enabled  id=['P0560']  x=9  y=10  input_suspected=on  indeterminate=off  increment_xy=on  downsample_count=1  ovr_cals=on  ovr_actions=on  show_actions=on  action1_name=''  action1_cond=(None)  action2_name=''  action2_cond=(None)  action3_name=''  action3_cond=(None)  action4_name=''  action4_cond=(None)
  wires:
  Unit Delay/1 -> Add/2
  Add/1 -> Abs/1
  Abs/1 -> Relational Operator/1
  motohawk_calibration4/1 -> Relational Operator/2
  Relational Operator/1 -> motohawk_fault_def2/1, Logical Operator2/1
  motohawk_calibration1/1 -> Relational Operator1/2
  Relational Operator1/1 -> motohawk_fault_def1/1, Logical Operator2/2
  motohawk_calibration2/1 -> Relational Operator2/2
  Relational Operator2/1 -> motohawk_fault_def3/1, Logical Operator2/3
  motohawk_ain/1 -> Product/1
  Constant/1 -> Product/2
  Product/1 -> Add/1, Unit Delay/1, Relational Operator1/1, Relational Operator2/1
  Logical Operator2/1 -> motohawk_fault_def4/1

== system Mooventure2016_Rev5/Foreground/Control/Faults/Power Train/Brake Pedal ==
  In1 : Inport
  Abs : Abs
  Add : Sum  Inputs=+-
  Bus Selector : BusSelector  OutputSignals=Driver Inputs.Brake_Position (signal 2)
  Bus Selector2 : BusSelector  OutputSignals=Driver Inputs.Brake_Position (signal 2)
  Bus Selector3 : BusSelector  OutputSignals=Driver Inputs.Brake_Position (signal 2)
  Bus Selector4 : BusSelector  OutputSignals=Driver Inputs.AgeCount (signal 1)
  Relational Operator : RelationalOperator  OutDataTypeStr=boolean
  Relational Operator2 : RelationalOperator  Operator=<=  OutDataTypeStr=boolean
  Relational Operator3 : RelationalOperator  OutDataTypeStr=boolean
  Relational Operator4 : RelationalOperator  OutDataTypeStr=boolean
  Unit Delay : UnitDelay  SampleTime=-1
  motohawk_calibration : MotoHawk_lib/Calibration & Probing Blocks/motohawk_calibration  nam='Brake_Pedal_Position_Intermiitent_Fault'  val=150  storage=Calibration  show_more=off  name_source=Use Parameter  data_type=Inherit from 'Default Value'  read_level=1  write_level=1  ovr_cals=on  view_as=Number  enum_struct={'Disabled', 'Enabled'}  vector_style=Wide Row  use_help_units=off  help=''  units=''  use_header_enum=off  row_header_enum={}  col_header_enum={}  use_min_max=off  min_val=-inf  max_val=inf  use_precision=off  precision=''  gain=1  offset=0  exp=1  use_mototune_group=off  mototune_group=motohawk_vardec_path(gcb)
  motohawk_calibration2 : MotoHawk_lib/Calibration & Probing Blocks/motohawk_calibration  nam='Brake_Pedal_Position_Low_Fault'  val=0  storage=Calibration  show_more=off  name_source=Use Parameter  data_type=Inherit from 'Default Value'  read_level=1  write_level=1  ovr_cals=on  view_as=Number  enum_struct={'Disabled', 'Enabled'}  vector_style=Wide Row  use_help_units=off  help=''  units=''  use_header_enum=off  row_header_enum={}  col_header_enum={}  use_min_max=off  min_val=-inf  max_val=inf  use_precision=off  precision=''  gain=1  offset=0  exp=1  use_mototune_group=off  mototune_group=motohawk_vardec_path(gcb)
  motohawk_calibration3 : MotoHawk_lib/Calibration & Probing Blocks/motohawk_calibration  nam='Brake_Pedal_Position_High_Fault'  val=33000  storage=Calibration  show_more=off  name_source=Use Parameter  data_type=Inherit from 'Default Value'  read_level=1  write_level=1  ovr_cals=on  view_as=Number  enum_struct={'Disabled', 'Enabled'}  vector_style=Wide Row  use_help_units=off  help=''  units=''  use_header_enum=off  row_header_enum={}  col_header_enum={}  use_min_max=off  min_val=-inf  max_val=inf  use_precision=off  precision=''  gain=1  offset=0  exp=1  use_mototune_group=off  mototune_group=motohawk_vardec_path(gcb)
  motohawk_calibration4 : MotoHawk_lib/Calibration & Probing Blocks/motohawk_calibration  nam='Brake_Pedal_Position_Communication_Loss_Fault'  val=1000  storage=Calibration  show_more=off  name_source=Use Parameter  data_type=Inherit from 'Default Value'  read_level=1  write_level=1  ovr_cals=on  view_as=Number  enum_struct={'Disabled', 'Enabled'}  vector_style=Wide Row  use_help_units=off  help=''  units=''  use_header_enum=off  row_header_enum={}  col_header_enum={}  use_min_max=off  min_val=-inf  max_val=inf  use_precision=off  precision=''  gain=1  offset=0  exp=1  use_mototune_group=off  mototune_group=motohawk_vardec_path(gcb)
  motohawk_fault_def1 : MotoHawk_lib/Fault Management Blocks/motohawk_fault_def  nam='Brake_Pedal_Position_Sensor_A_Circuit_High'  mode=Enabled  id=['P1532']  x=1000  y=2000  input_suspected=on  indeterminate=off  increment_xy=on  downsample_count=1  ovr_cals=on  ovr_actions=on  show_actions=on  action1_name='Wrench_Light'  action1_cond=Active  action2_name=''  action2_cond=(None)  action3_name=''  action3_cond=(None)  action4_name=''  action4_cond=(None)
  motohawk_fault_def2 : MotoHawk_lib/Fault Management Blocks/motohawk_fault_def  nam='Brake_Pedal_Position_Intermiitent'  mode=Enabled  id=['P1530']  x=9  y=10  input_suspected=on  indeterminate=off  increment_xy=on  downsample_count=1  ovr_cals=on  ovr_actions=on  show_actions=on  action1_name='Wrench_Light'  action1_cond=Active  action2_name=''  action2_cond=(None)  action3_name=''  action3_cond=(None)  action4_name=''  action4_cond=(None)
  motohawk_fault_def4 : MotoHawk_lib/Fault Management Blocks/motohawk_fault_def  nam='Brake_Pedal_Position_Low'  mode=Enabled  id=['P1531']  x=5  y=10  input_suspected=on  indeterminate=off  increment_xy=on  downsample_count=1  ovr_cals=on  ovr_actions=on  show_actions=on  action1_name='Wrench_Light'  action1_cond=Active  action2_name=''  action2_cond=(None)  action3_name=''  action3_cond=(None)  action4_name=''  action4_cond=(None)
  motohawk_fault_def5 : MotoHawk_lib/Fault Management Blocks/motohawk_fault_def  nam='Brake_Pedal_Position_Communication_Loss'  mode=Enabled  id=['P1533']  x=5  y=10  input_suspected=on  indeterminate=off  increment_xy=on  downsample_count=1  ovr_cals=on  ovr_actions=on  show_actions=on  action1_name='Wrench_Light'  action1_cond=Active  action2_name='Regen_Brakes_Disabled'  action2_cond=Active  action3_name=''  action3_cond=(None)  action4_name=''  action4_cond=(None)
  wires:
  In1/1 -> Bus Selector/1, Bus Selector2/1, Bus Selector3/1, Bus Selector4/1
  Bus Selector/1 -> Add/1, Unit Delay/1  "<Brake_Position (signal 2)>"
  Unit Delay/1 -> Add/2
  Add/1 -> Abs/1
  Abs/1 -> Relational Operator/1
  Relational Operator/1 -> motohawk_fault_def2/1
  motohawk_calibration/1 -> Relational Operator/2
  motohawk_calibration2/1 -> Relational Operator2/2
  Relational Operator2/1 -> motohawk_fault_def4/1
  Bus Selector3/1 -> Relational Operator3/1  "<Brake_Position (signal 2)>"
  motohawk_calibration3/1 -> Relational Operator3/2
  Relational Operator3/1 -> motohawk_fault_def1/1
  Bus Selector2/1 -> Relational Operator2/1  "<Brake_Position (signal 2)>"
  Bus Selector4/1 -> Relational Operator4/1  "<AgeCount (signal 1)>"
  motohawk_calibration4/1 -> Relational Operator4/2
  Relational Operator4/1 -> motohawk_fault_def5/1

== system Mooventure2016_Rev5/Foreground/Control/Faults/Power Train/Cruise Control ==
  In1 : Inport
  Bus Selector : BusSelector  OutputSignals=Cruise Control.ON,Cruise Control.Off,Cruise Control.RSM,Cruise Control.Set+,Cruise Control.Set-
  Bus Selector1 : BusSelector  OutputSignals=Driver Inputs.Brake_Position (signal 2)
  Bus Selector2 : BusSelector  OutputSignals=Driver Inputs.Brake_Position (signal 2)
  Data Type Conversion{,1..4} (5 alike) : DataTypeConversion  OutDataTypeStr=boolean
  Detect Change{,1..4} (5 alike) : simulink/Logic and Bit Operations/Detect Change  SystemSampleTime=-1  vinit=0
  Logical Operator2 : Logic  Operator=OR  AllPortsSameDT=off  OutDataTypeStr=boolean
  Relational Operator1 : RelationalOperator  Operator=>  OutDataTypeStr=boolean
  Relational Operator2 : RelationalOperator  Operator=<=  OutDataTypeStr=boolean
  motohawk_calibration1 : MotoHawk_lib/Calibration & Probing Blocks/motohawk_calibration  nam='Cruise_Disable_Brake_Fault2'  val=0  storage=Calibration  show_more=off  name_source=Use Parameter  data_type=Inherit from 'Default Value'  read_level=1  write_level=1  ovr_cals=on  view_as=Number  enum_struct={'Disabled', 'Enabled'}  vector_style=Wide Row  use_help_units=off  help=''  units=''  use_header_enum=off  row_header_enum={}  col_header_enum={}  use_min_max=off  min_val=-inf  max_val=inf  use_precision=off  precision=''  gain=1  offset=0  exp=1  use_mototune_group=off  mototune_group=motohawk_vardec_path(gcb)
  motohawk_calibration2 : MotoHawk_lib/Calibration & Probing Blocks/motohawk_calibration  nam='Cruise_Disable_Brake_Fault1'  val=33000  storage=Calibration  show_more=off  name_source=Use Parameter  data_type=Inherit from 'Default Value'  read_level=1  write_level=1  ovr_cals=on  view_as=Number  enum_struct={'Disabled', 'Enabled'}  vector_style=Wide Row  use_help_units=off  help=''  units=''  use_header_enum=off  row_header_enum={}  col_header_enum={}  use_min_max=off  min_val=-inf  max_val=inf  use_precision=off  precision=''  gain=1  offset=0  exp=1  use_mototune_group=off  mototune_group=motohawk_vardec_path(gcb)
  motohawk_fault_def1 : MotoHawk_lib/Fault Management Blocks/motohawk_fault_def  nam='Cruise_Control_Off_Signal_Malfunction'  mode=Enabled  id=['P0566']  x=5  y=10  input_suspected=on  indeterminate=off  increment_xy=on  downsample_count=1  ovr_cals=on  ovr_actions=on  show_actions=on  action1_name='Wrench_Light'  action1_cond=Active  action2_name='Cruise'  action2_cond=Active  action3_name=''  action3_cond=(None)  action4_name=''  action4_cond=(None)
  motohawk_fault_def2 : MotoHawk_lib/Fault Management Blocks/motohawk_fault_def  nam='Cruise_Control_Resume_Signal_Malfunction'  mode=Enabled  id=['P0567']  x=5  y=10  input_suspected=on  indeterminate=off  increment_xy=on  downsample_count=1  ovr_cals=on  ovr_actions=on  show_actions=on  action1_name='Wrench_Light'  action1_cond=Active  action2_name='Cruise'  action2_cond=Active  action3_name=''  action3_cond=(None)  action4_name=''  action4_cond=(None)
  motohawk_fault_def3 : MotoHawk_lib/Fault Management Blocks/motohawk_fault_def  nam='Cruise_Control_Set_Signal_Malfunction'  mode=Enabled  id=['P0568']  x=15  y=20  input_suspected=on  indeterminate=off  increment_xy=on  downsample_count=1  ovr_cals=on  ovr_actions=on  show_actions=on  action1_name='Wrench_Light'  action1_cond=Active  action2_name='Cruise'  action2_cond=Active  action3_name=''  action3_cond=(None)  action4_name=''  action4_cond=(None)
  motohawk_fault_def4 : MotoHawk_lib/Fault Management Blocks/motohawk_fault_def  nam='Cruise_Control_Coast_Signal_Malfunction'  mode=Enabled  id=['P0569']  x=15  y=20  input_suspected=on  indeterminate=off  increment_xy=on  downsample_count=1  ovr_cals=on  ovr_actions=on  show_actions=on  action1_name='Wrench_Light'  action1_cond=Active  action2_name='Cruise'  action2_cond=Active  action3_name=''  action3_cond=(None)  action4_name=''  action4_cond=(None)
  motohawk_fault_def5 : MotoHawk_lib/Fault Management Blocks/motohawk_fault_def  nam='Cruise_Control_Brake_Switch_A_Circuit_High'  mode=Enabled  id=['P0573']  x=15  y=20  input_suspected=on  indeterminate=off  increment_xy=on  downsample_count=1  ovr_cals=on  ovr_actions=on  show_actions=on  action1_name='Wrench_Light'  action1_cond=Active  action2_name='Cruise'  action2_cond=Active  action3_name=''  action3_cond=(None)  action4_name=''  action4_cond=(None)
  motohawk_fault_def6 : MotoHawk_lib/Fault Management Blocks/motohawk_fault_def  nam='Cruise_Control_Brake_Switch_A_Circuit_Low'  mode=Enabled  id=['P0572']  x=15  y=20  input_suspected=on  indeterminate=off  increment_xy=on  downsample_count=1  ovr_cals=on  ovr_actions=on  show_actions=on  action1_name='Wrench_Light'  action1_cond=Active  action2_name='Cruise'  action2_cond=Active  action3_name=''  action3_cond=(None)  action4_name=''  action4_cond=(None)
  motohawk_fault_def7 : MotoHawk_lib/Fault Management Blocks/motohawk_fault_def  nam='Cruise_Control_Brake_Switch_A_Circuit_Malfunction'  mode=Enabled  id=['P0571']  x=9  y=10  input_suspected=on  indeterminate=off  increment_xy=on  downsample_count=1  ovr_cals=on  ovr_actions=on  show_actions=on  action1_name=''  action1_cond=(None)  action2_name=''  action2_cond=(None)  action3_name=''  action3_cond=(None)  action4_name=''  action4_cond=(None)
  motohawk_fault_def8 : MotoHawk_lib/Fault Management Blocks/motohawk_fault_def  nam='Cruise_Control_On_Signal_Malfunction'  mode=Enabled  id=['P0565']  x=5  y=10  input_suspected=on  indeterminate=off  increment_xy=on  downsample_count=1  ovr_cals=on  ovr_actions=on  show_actions=on  action1_name='Wrench_Light'  action1_cond=Active  action2_name='Cruise'  action2_cond=Active  action3_name=''  action3_cond=(None)  action4_name=''  action4_cond=(None)
  motohawk_fault_status : MotoHawk_lib/Fault Management Blocks/motohawk_fault_status  source=Lookup By Name  nam='Cruise_Control_Brake_Switch_A_Circuit_High'  status=Active
  motohawk_fault_status1 : MotoHawk_lib/Fault Management Blocks/motohawk_fault_status  source=Lookup By Name  nam='Cruise_Control_Brake_Switch_A_Circuit_Low'  status=Active
  wires:
  In1/1 -> Bus Selector/1, Bus Selector1/1, Bus Selector2/1
  Bus Selector/1 -> Detect Change/1  "<ON>"
  Bus Selector/2 -> Detect Change1/1  "<Off>"
  Bus Selector/3 -> Detect Change2/1  "<RSM>"
  Bus Selector/4 -> Detect Change3/1  "<Set+>"
  Bus Selector/5 -> Detect Change4/1  "<Set->"
  Detect Change/1 -> Data Type Conversion/1
  Detect Change1/1 -> Data Type Conversion1/1
  Detect Change2/1 -> Data Type Conversion2/1
  Detect Change3/1 -> Data Type Conversion3/1
  Detect Change4/1 -> Data Type Conversion4/1
  Bus Selector1/1 -> Relational Operator1/1  "<Brake_Position (signal 2)>"
  motohawk_calibration2/1 -> Relational Operator1/2
  Relational Operator1/1 -> motohawk_fault_def5/1
  Bus Selector2/1 -> Relational Operator2/1  "<Brake_Position (signal 2)>"
  motohawk_calibration1/1 -> Relational Operator2/2
  Relational Operator2/1 -> motohawk_fault_def6/1
  motohawk_fault_status1/1 -> Logical Operator2/2
  motohawk_fault_status/1 -> Logical Operator2/1
  Logical Operator2/1 -> motohawk_fault_def7/1
  Data Type Conversion/1 -> motohawk_fault_def8/1
  Data Type Conversion1/1 -> motohawk_fault_def1/1
  Data Type Conversion2/1 -> motohawk_fault_def2/1
  Data Type Conversion3/1 -> motohawk_fault_def3/1
  Data Type Conversion4/1 -> motohawk_fault_def4/1
